simulink model "SCmodulator"  (R2024b)
settings: Solver=FixedStepDiscrete  StartTime=0.0  StopTime=10.0  RelTol=1e-3
undefined symbols (not defined in the file): const_16APSK, FXP, SC, sysParams
libraries: dspmlti4 x2, hdlsllib x2, commdigbbndpm3 x1, commdigbbndam3 x1
settings Model: DataTypeOverride=Off  Creator=aless  LastModifiedBy=aless
settings SolverCC: PositivePriorityOrder=on
settings OptimizationCC: BlockReduction=off  ConditionallyExecuteInputs=off  DefaultParameterBehavior=Inlined  InheritOutputTypeSmallerThanSingle=on  EnhancedBackFolding=on  PassReuseOutputArgsAs=Individual arguments  ZeroExternalMemoryAtStartup=off  ZeroInternalMemoryAtStartup=off  MaxStackSize=64  OptimizeBlockOrder=speed  DifferentSizesBufferReuse=on  OptimizationCustomize=off  EfficientTunableParamExpr=on
settings DebuggingCC: AlgebraicLoopMsg=error  SingleTaskRateTransMsg=error  ParameterTunabilityLossMsg=error  UnconnectedInputMsg=warning  UnconnectedOutputMsg=warning  UnconnectedLineMsg=warning
settings HardwareCC: ProdBitPerPointer=32  ProdBitPerSizeT=32  ProdBitPerPtrDiffT=32  ProdLargestAtomicFloat=None  ProdIntDivRoundTo=Undefined  ProdEndianess=Unspecified  ProdWordSize=32  ProdHWDeviceType=ASIC/FPGA->ASIC/FPGA  TargetBitPerPointer=64  TargetBitPerSizeT=64  TargetBitPerPtrDiffT=64  TargetLongLongMode=on  TargetIntDivRoundTo=Zero  TargetEndianess=LittleEndian  TargetWordSize=64  TargetHWDeviceType=Custom Processor->MATLAB Host Computer  ProdEqTarget=off  HardwareBoardFeatureSet=SoCBlockset
settings ModelReferenceCC: ModelReferenceNumInstancesAllowed=Single
settings RTWCC: Description=Embedded Coder  SystemTargetFile=ert.tlc  HardwareBoard=Xilinx Zynq UltraScale+ RFSoC ZCU208 Evaluation Kit  TLCOptions="-aInlineSetEventsForThisBaseRateFcn=TLC_FALSE -aSuppressMultiTaskScheduler=TLC_FALSE  -aRateBasedStepFcn=0"  TemplateMakefile=ert_default_tmf  Toolchain=Linaro AArch64 Linux v6.3.1
settings CodeAppCC: ForceParamTrailComments=on  IgnoreCustomStorageClasses=off  OperatorAnnotations=on  SimulinkDataObjDesc=on  SFDataObjDesc=on  InsertBlockDesc=on

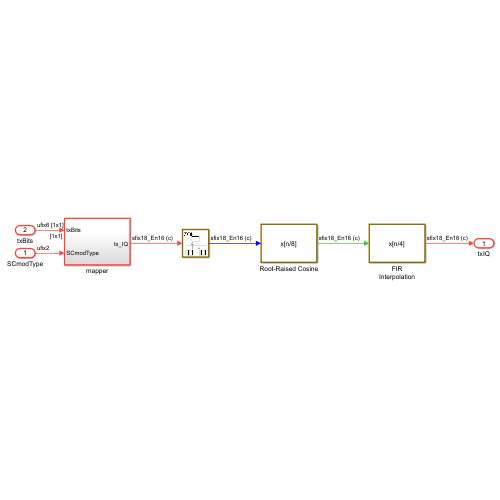
[thumbnail: Simulink's stored preview of the top-level diagram]
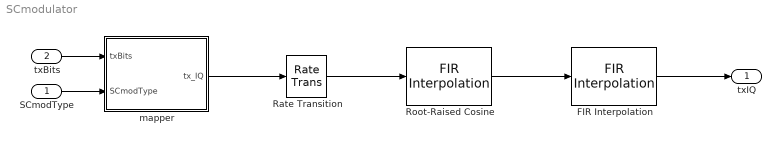
== system SCmodulator ==
  SCmodType : Inport  OutDataTypeStr=fixdt(0,2,0)  SampleTime=sysParams.FPGAClkPeriod
  txBits : Inport  Port=2  OutDataTypeStr=fixdt(0,6,0)  SampleTime=sysParams.FPGAClkPeriod
  FIR Interpolation : dspmlti4/FIR Interpolation  FilterSource=Dialog parameters  PrivateCoeffs=0  h=SC.firTaps  L=SC.firInterpFactor  FilterObject=FINTERP  framing=Allow multirate processing  outputBufInitCond=0  roundingMode=Floor  overflowMode=off  firstCoeffMode=Binary point scaling  firstCoeffWordLength=FXP.coeffWL  firstCoeffFracLength=FXP.coeffFL  firstCoeffDataTypeStr=fixdt(1,FXP.coeffWL,FXP.coeffFL)  firstCoeffMin=[]  firstCoeffMax=[]  firstCoeffLastDataTypeStr=fixdt(1,FXP.coeffWL,FXP.coeffFL)  outputMode=Binary point scaling  outputWordLength=FXP.sampWL  outputFracLength=FXP.sampFL  outputDataTypeStr=fixdt(1,FXP.sampWL,FXP.sampFL)  outputMin=[]  outputMax=[]  outputLastDataTypeStr=fixdt(1,FXP.sampWL,FXP.sampFL)
  Rate Transition : RateTransition  OutPortSampleTimeMultiple=40  OutPortSampleTime=1/SC.symRate
  Root-Raised Cosine : dspmlti4/FIR Interpolation  FilterSource=Dialog parameters  PrivateCoeffs=0  h=SC.RRC.taps  L=SC.RRC.sampPerSym  FilterObject=FINTERP  framing=Allow multirate processing  outputBufInitCond=0  roundingMode=Floor  overflowMode=off  firstCoeffMode=Binary point scaling  firstCoeffWordLength=FXP.coeffWL  firstCoeffFracLength=FXP.coeffFL  firstCoeffDataTypeStr=fixdt(1,FXP.coeffWL,FXP.coeffFL)  firstCoeffMin=[]  firstCoeffMax=[]  firstCoeffLastDataTypeStr=fixdt(1,FXP.coeffWL,FXP.coeffFL)  outputMode=Binary point scaling  outputWordLength=FXP.sampWL  outputFracLength=FXP.sampFL  outputDataTypeStr=fixdt(1,FXP.sampWL,FXP.sampFL)  outputMin=[]  outputMax=[]  outputLastDataTypeStr=fixdt(1,FXP.sampWL,FXP.sampFL)
  mapper : Subsystem
  txIQ : Outport
  wires:
  mapper/1(tx_IQ) -> Rate Transition/1
  Rate Transition/1 -> Root-Raised Cosine/1
  txBits/1 -> mapper/1(txBits)
  Root-Raised Cosine/1 -> FIR Interpolation/1
  FIR Interpolation/1 -> txIQ/1
  SCmodType/1 -> mapper/2(SCmodType)

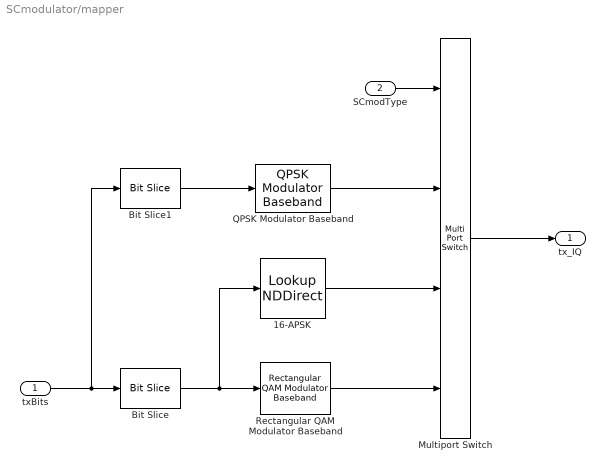
== system SCmodulator/mapper ==
  txBits : Inport
  SCmodType : Inport  Port=2
  16-APSK : LookupNDDirect  NumberOfTableDimensions=1  Table=const_16APSK  DiagnosticForOutOfRangeInput=Error  TableDataTypeStr=fixdt(1,FXP.sampWL,FXP.sampFL)
  Bit Slice : hdlsllib/Logic and Bit Operations/Bit Slice  lidx=3  ridx=0
  Bit Slice1 : hdlsllib/Logic and Bit Operations/Bit Slice  lidx=1  ridx=0
  Multiport Switch : MultiPortSwitch  DataPortOrder=Zero-based contiguous  zeroidx=on  OutDataTypeStr=fixdt(1,FXP.sampWL,FXP.sampFL)  SaturateOnIntegerOverflow=off  InputSameDT=off
  QPSK Modulator Baseband : commdigbbndpm3/QPSK Modulator Baseband  InType=Integer  Enc=Gray  Ph=pi/4  outDtype=Fixed-point  outWordLen=FXP.sampWL  outUDDataType=sfix(16)  outFracLenMode=User-defined  outFracLen=FXP.sampFL  outDataTypeStr=fixdt(1,FXP.sampWL,FXP.sampFL)  outLastDataTypeStr=fixdt(1,FXP.sampWL,FXP.sampFL)
  Rectangular QAM Modulator Baseband : commdigbbndam3/Rectangular QAM Modulator Baseband  M=16  InType=Integer  Enc=Gray  Mapping=[0:15]  PowType=Average Power  MinDist=2  AvgPow=1  PeakPow=1  Ph=0  outDtype=Fixed-point  outWordLen=FXP.sampWL  outUDDataType=sfix(16)  outFracLenMode=User-defined  outFracLen=FXP.sampFL  outDataTypeStr=fixdt(1,FXP.sampWL,FXP.sampFL)  outLastDataTypeStr=fixdt(1,FXP.sampWL,FXP.sampFL)
  tx_IQ : Outport
  wires:
  Bit Slice1/1 -> QPSK Modulator Baseband/1
  Bit Slice/1 -> 16-APSK/1, Rectangular QAM Modulator Baseband/1
  txBits/1 -> Bit Slice1/1, Bit Slice/1
  QPSK Modulator Baseband/1 -> Multiport Switch/2
  Rectangular QAM Modulator Baseband/1 -> Multiport Switch/4
  SCmodType/1 -> Multiport Switch/1
  Multiport Switch/1 -> tx_IQ/1
  16-APSK/1 -> Multiport Switch/3
